simulink model "week5_inclass_stanley"  (R2020b)
settings: Solver=FixedStepAuto  StartTime=0.0  StopTime=Ts  FixedStep=0.1  MaxStep=1e-2  RelTol=1e-3  AbsTol=1e-3
InitFcn:
  | stanley_init
StopFcn:
  | simulation_plots_week5
undefined symbols (not defined in the file or in its folder): vRef
libraries: autolibshared x1, simulink_extras x1, drivingvehiclecontroller x1
settings Model: Creator=anime  LastModifiedBy=anime

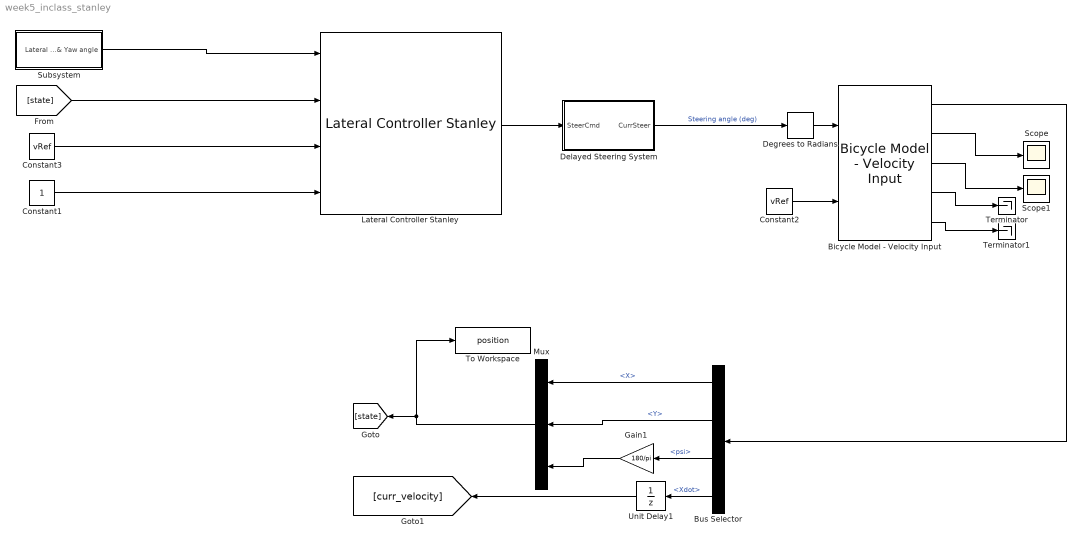
== system week5_inclass_stanley ==
  Bicycle Model - Velocity Input : autolibshared/Bicycle Model - Velocity Input  trackMode=Single (bicycle)  inputMode=External longitudinal forces  frontSteerMode=on  rearSteerMode=off  windMode=off  muMode=off  extFMode=off  extMMode=off  aMode=3  NF=2  NR=2  m=1575  a=1.2  b=1.6  h=0.35  X_o=X_o  xdot_o=0  CalphaMode=off  sigmaMode=on  w=[1.4,1.4]  Cy_f=19e3  Cy_r=20e3  sigma_f=.1  sigma_r=.1  alpha_f_brk=[-.1 .1]  Cy_f_data=[-9e3 9e3]  alpha_r_brk=[-.1 .1]  Cy_r_data=[-9e3 9e3]  Y_o=Y_o  ydot_o=0  Izz=4000  psi_o=psi_o  r_o=0  Af=2  Cd=.3  Cl=.1  Cpm=.1  beta_w=[0:0.01:0.3]  Cs=[0:0.03:0.9]  Cym=[0:0.01:0.3]  Pabs=101325  Tair=273  g=9.81  mu=1  xdot_tol=.01  Fznom=5000  Fxtire_sat=1e6  Fytire_sat=1e6  longOff=0  latOff=0  vertOff=0
      settings: SourceProductBaseCode=PW,MT,UV,VE,VP
  Bus Selector : BusSelector  OutputSignals=InertFrm.Cg.Disp.X,InertFrm.Cg.Disp.Y,InertFrm.Cg.Ang.psi,InertFrm.Cg.Vel.Xdot
  Constant1 : Constant
  Constant2 : Constant  Value=vRef
  Constant3 : Constant  Value=vRef
  Degrees to Radians : simulink_extras/Transformations/Degrees to Radians
      settings: SourceProductName=Simulink Extras
  Delayed Steering System : Subsystem
  Gain1 : Gain  Gain=180/pi
  Lateral Controller Stanley : drivingvehiclecontroller/Lateral Controller Stanley  ModelType=Kinematic bicycle model  PositionGainF=K  PositionGainR=1  YawRateGain=0.2  DelayGain=0.2  VehicleMass=1575  Lf=1.2  Lr=1.6  TireStiffness=19000  Wheelbase=L  MaxSteeringAngle=35
      settings: SourceProductBaseCode=DR
  Mux : Mux  Inputs=3
  Scope : Scope
  Scope1 : Scope
  Subsystem : Subsystem
  Terminator : Terminator
  Terminator1 : Terminator
  To Workspace : ToWorkspace  VariableName=position  SampleTime=-1
  Unit Delay1 : UnitDelay  InitialCondition=vRef  SampleTime=-1  HasFrameUpgradeWarning=on
  wires:
  Constant1/1 -> Lateral Controller Stanley/4
  Mux/1 -> To Workspace/1, [state]
  Lateral Controller Stanley/1 -> Delayed Steering System/1(SteerCmd)
  Bus Selector/1 -> Mux/1  "<X>"
  Bus Selector/3 -> Gain1/1  "<psi>"
  Bicycle Model - Velocity Input/5 -> Terminator1/1
  Bicycle Model - Velocity Input/1 -> Bus Selector/1
  Bicycle Model - Velocity Input/4 -> Terminator/1
  Bus Selector/2 -> Mux/2  "<Y>"
  Bicycle Model - Velocity Input/3 -> Scope1/1
  Bicycle Model - Velocity Input/2 -> Scope/1
  [state] -> Lateral Controller Stanley/2
  Subsystem/1(Lateral position & Yaw angle) -> Lateral Controller Stanley/1
  Constant2/1 -> Bicycle Model - Velocity Input/2
  Delayed Steering System/1(CurrSteer) -> Degrees to Radians/1  "Steering angle (deg)"
  Degrees to Radians/1 -> Bicycle Model - Velocity Input/1
  Gain1/1 -> Mux/3
  Bus Selector/4 -> Unit Delay1/1  "<Xdot>"
  Unit Delay1/1 -> [curr_velocity]
  Constant3/1 -> Lateral Controller Stanley/3

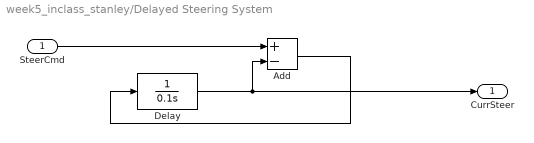
== system week5_inclass_stanley/Delayed Steering System ==
  SteerCmd : Inport
  Add : Sum  Inputs=+-
  Delay : TransferFcn  Denominator=[0.1 0]
  CurrSteer : Outport  VectorParamsAs1DForOutWhenUnconnected=off
  wires:
  Add/1 -> Delay/1
  SteerCmd/1 -> Add/1
  Delay/1 -> CurrSteer/1, Add/2

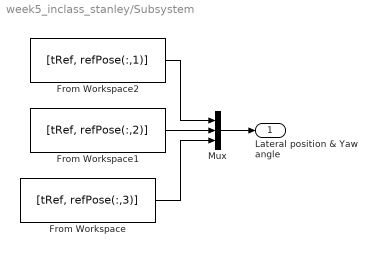
== system week5_inclass_stanley/Subsystem ==
  From Workspace : FromWorkspace  VariableName=[tRef, refPose(:,3)]  SampleTime=0.1
  From Workspace1 : FromWorkspace  VariableName=[tRef, refPose(:,2)]  SampleTime=0.1
  From Workspace2 : FromWorkspace  VariableName=[tRef, refPose(:,1)]  SampleTime=0.1
  Mux : Mux  Inputs=3
  Lateral position & Yaw angle : Outport  VectorParamsAs1DForOutWhenUnconnected=off
  wires:
  From Workspace2/1 -> Mux/1
  Mux/1 -> Lateral position & Yaw angle/1
  From Workspace/1 -> Mux/3
  From Workspace1/1 -> Mux/2
